simulink model "pancreas"  (R2019a)
settings: Solver=VariableStepAuto  StartTime=0.0  StopTime=200  RelTol=1e-3
model workspace (MAT data in the model file):
  K = 0.00794
  N1 = 0.00747
  N2 = 0.0958
  a = 0.0482
  b = 0.931
  lambda = 0.0958
settings Model: Creator=rache  LastModifiedBy=rache
settings DataIOCC: ReturnWorkspaceOutputs=off
settings DebuggingCC: ArithmeticOperatorsInVariantConditions=warning

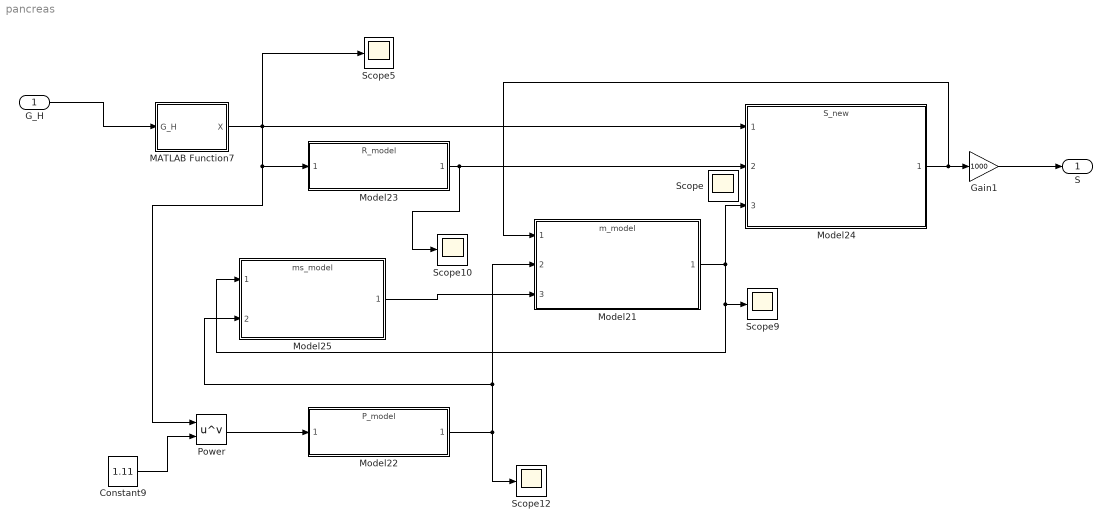
== system pancreas ==
  G_H : Inport
  Constant9 : Constant  Value=1.11
  Gain1 : Gain  Gain=1000
  MATLAB Function7 : MATLAB Function  TreatAsAtomicUnit=on
  Model21 : ModelReference  ModelNameDialog=m_model  SimulationMode=Normal  ModelReferenceVersion=1.10
  Model22 : ModelReference  ModelNameDialog=P_model  SimulationMode=Normal  ModelReferenceVersion=1.10
  Model23 : ModelReference  ModelNameDialog=R_model.slx  SimulationMode=Normal  ModelReferenceVersion=1.8
  Model24 : ModelReference  ModelNameDialog=S_new  SimulationMode=Normal  ModelReferenceVersion=1.4
  Model25 : ModelReference  ModelNameDialog=ms_model  SimulationMode=Normal  ModelReferenceVersion=1.8
  Power : Math  Operator=pow  SaturateOnIntegerOverflow=on
  Scope{,5,9..10,12} (5 alike) : Scope
  S : Outport  OutMin=0
  wires:
  Model24/1 -> Gain1/1, Model21/1
  Model22/1 -> Model21/2, Model25/2, Scope12/1
  Model25/1 -> Model21/3
  Model21/1 -> Model25/1, Scope9/1, Model24/3
  MATLAB Function7/1(X) -> Scope5/1, Power/1, Model23/1, Model24/1
  Model23/1 -> Scope10/1, Model24/2
  Constant9/1 -> Power/2
  Power/1 -> Model22/1
  G_H/1 -> MATLAB Function7/1(G_H)
  Gain1/1 -> S/1

== matlab function pancreas/MATLAB Function7 ==
  data: G_H input; X output
function X = X_function(G_H)
%X_FUNCTION Calculate X from G_H (glucose output of heart)
%   Inputs: G_H (g)
%   Outputs: X (glucose enhanced excitation factor)
num = G_H^3.27;
denom = (132^3.27 + 5.93*((G_H)^3.02));
X = num/denom;
end
